simulink model "problem1_robotsim"  (R2021a)
settings: Solver=FixedStepAuto  StartTime=0.0  StopTime=tstop  FixedStep=1e-3  MaxStep=1e-2
values from neighbouring files (symbols this model uses):
  f_v = [0.1 0.1 0.1 0.05 0.05 0.05]'    [problem1.m]    (also in problem3.m = zeros(6,1))
  fext = zeros(6,8)    [problem1.m]    (also in problem3.m)
  qdotinit = zeros(6,1)    [problem1.m]    (also in problem3.m)
  qinit = zeros(6,1)    [problem1.m]    (also in problem3.m)
  tau = zeros(6,1)    [problem1.m]    (also in problem3.m)
libraries: simulink x1, robotmaniplib x1
settings Model: Creator=wen  LastModifiedBy=Eric Tung
settings SolverCC: AlgebraicLoopSolver=TrustRegion
settings DebuggingCC: SFMachineParentedDataDiag=warning

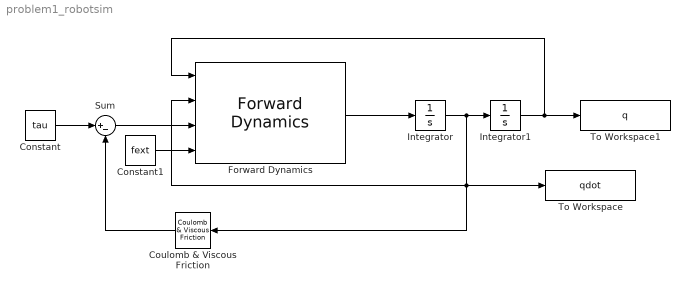
== system problem1_robotsim ==
  Constant : Constant  Value=tau
  Constant1 : Constant  Value=fext
  Coulomb & Viscous Friction : simulink/Discontinuities/Coulomb & Viscous Friction  offset=f_c  gain=f_v
  Forward Dynamics : robotmaniplib/Forward Dynamics  RigidBodyTree=abb  SimulateUsing=Interpreted execution
  Integrator : Integrator  InitialCondition=qdotinit
  Integrator1 : Integrator  InitialCondition=qinit
  Sum : Sum  Inputs=|+-
  To Workspace : ToWorkspace  VariableName=qdot  SampleTime=-1
  To Workspace1 : ToWorkspace  VariableName=q  SampleTime=-1
  wires:
  Forward Dynamics/1 -> Integrator/1
  Integrator/1 -> Coulomb & Viscous Friction/1, Forward Dynamics/2, To Workspace/1, Integrator1/1
  Integrator1/1 -> Forward Dynamics/1, To Workspace1/1
  Constant1/1 -> Forward Dynamics/4
  Coulomb & Viscous Friction/1 -> Sum/2
  Sum/1 -> Forward Dynamics/3
  Constant/1 -> Sum/1
